simulink model "output_buffer"  (R2016b)
settings: Solver=VariableStepAuto  StartTime=0.0  StopTime=5000  RelTol=1e-3
undefined symbols (not defined in the file or in its folder): fft_stages, output_len_bits
libraries: xbsIndex_r4 x750, casper_library_misc x6, simulink x2
(part 3 of 3)

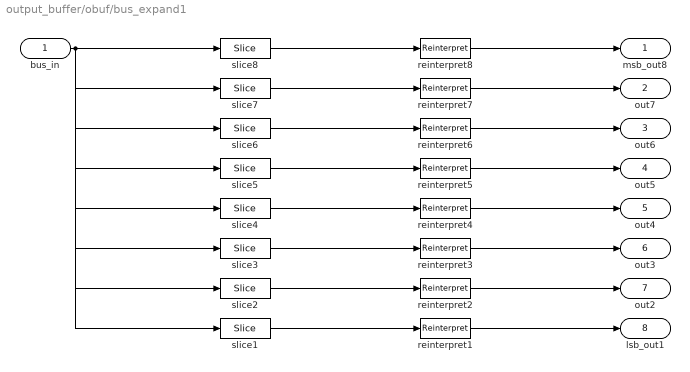
== system output_buffer/obuf/bus_expand1 ==
  bus_in : Inport
  reinterpret{1..8} (8 alike) : xbsIndex_r4/Reinterpret  force_arith_type=on  arith_type=Unsigned  force_bin_pt=on  bin_pt=0  block_type=reinterpret
  slice1 : xbsIndex_r4/Slice  nbits=32  boolean_output=off  mode=Upper Bit Location + Width  bit1=-224  base1=MSB of Input  bit0=0  base0=LSB of Input  dbl_ovrd=off  block_type=slice
  slice2 : xbsIndex_r4/Slice  nbits=32  boolean_output=off  mode=Upper Bit Location + Width  bit1=-192  base1=MSB of Input  bit0=0  base0=LSB of Input  dbl_ovrd=off  block_type=slice
  slice3 : xbsIndex_r4/Slice  nbits=32  boolean_output=off  mode=Upper Bit Location + Width  bit1=-160  base1=MSB of Input  bit0=0  base0=LSB of Input  dbl_ovrd=off  block_type=slice
  slice4 : xbsIndex_r4/Slice  nbits=32  boolean_output=off  mode=Upper Bit Location + Width  bit1=-128  base1=MSB of Input  bit0=0  base0=LSB of Input  dbl_ovrd=off  block_type=slice
  slice5 : xbsIndex_r4/Slice  nbits=32  boolean_output=off  mode=Upper Bit Location + Width  bit1=-96  base1=MSB of Input  bit0=0  base0=LSB of Input  dbl_ovrd=off  block_type=slice
  slice6 : xbsIndex_r4/Slice  nbits=32  boolean_output=off  mode=Upper Bit Location + Width  bit1=-64  base1=MSB of Input  bit0=0  base0=LSB of Input  dbl_ovrd=off  block_type=slice
  slice7 : xbsIndex_r4/Slice  nbits=32  boolean_output=off  mode=Upper Bit Location + Width  bit1=-32  base1=MSB of Input  bit0=0  base0=LSB of Input  dbl_ovrd=off  block_type=slice
  slice8 : xbsIndex_r4/Slice  nbits=32  boolean_output=off  mode=Upper Bit Location + Width  bit1=0  base1=MSB of Input  bit0=0  base0=LSB of Input  dbl_ovrd=off  block_type=slice
  msb_out8 : Outport
  out7 : Outport  Port=2
  out6 : Outport  Port=3
  out5 : Outport  Port=4
  out4 : Outport  Port=5
  out3 : Outport  Port=6
  out2 : Outport  Port=7
  lsb_out1 : Outport  Port=8
  wires:
  bus_in/1 -> slice8/1, slice7/1, slice6/1, slice5/1, slice4/1, slice3/1, slice2/1, slice1/1
  slice8/1 -> reinterpret8/1
  reinterpret8/1 -> msb_out8/1
  slice7/1 -> reinterpret7/1
  reinterpret7/1 -> out7/1
  slice6/1 -> reinterpret6/1
  reinterpret6/1 -> out6/1
  slice5/1 -> reinterpret5/1
  reinterpret5/1 -> out5/1
  slice4/1 -> reinterpret4/1
  reinterpret4/1 -> out4/1
  slice3/1 -> reinterpret3/1
  reinterpret3/1 -> out3/1
  slice2/1 -> reinterpret2/1
  reinterpret2/1 -> out2/1
  slice1/1 -> reinterpret1/1
  reinterpret1/1 -> lsb_out1/1

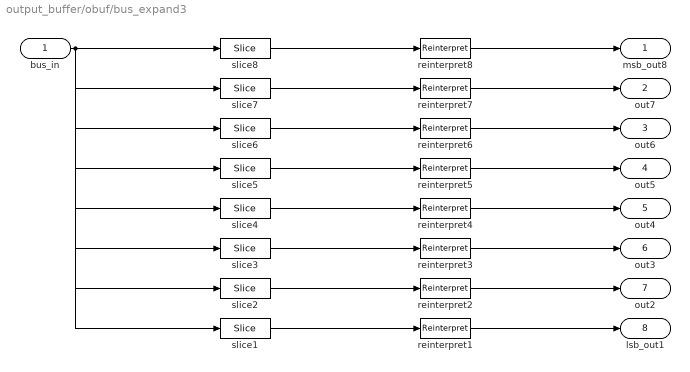
== system output_buffer/obuf/bus_expand3 ==
  bus_in : Inport
  reinterpret{1..8} (8 alike) : xbsIndex_r4/Reinterpret  force_arith_type=on  arith_type=Unsigned  force_bin_pt=on  bin_pt=0  block_type=reinterpret
  slice1 : xbsIndex_r4/Slice  nbits=32  boolean_output=off  mode=Upper Bit Location + Width  bit1=-224  base1=MSB of Input  bit0=0  base0=LSB of Input  dbl_ovrd=off  block_type=slice
  slice2 : xbsIndex_r4/Slice  nbits=32  boolean_output=off  mode=Upper Bit Location + Width  bit1=-192  base1=MSB of Input  bit0=0  base0=LSB of Input  dbl_ovrd=off  block_type=slice
  slice3 : xbsIndex_r4/Slice  nbits=32  boolean_output=off  mode=Upper Bit Location + Width  bit1=-160  base1=MSB of Input  bit0=0  base0=LSB of Input  dbl_ovrd=off  block_type=slice
  slice4 : xbsIndex_r4/Slice  nbits=32  boolean_output=off  mode=Upper Bit Location + Width  bit1=-128  base1=MSB of Input  bit0=0  base0=LSB of Input  dbl_ovrd=off  block_type=slice
  slice5 : xbsIndex_r4/Slice  nbits=32  boolean_output=off  mode=Upper Bit Location + Width  bit1=-96  base1=MSB of Input  bit0=0  base0=LSB of Input  dbl_ovrd=off  block_type=slice
  slice6 : xbsIndex_r4/Slice  nbits=32  boolean_output=off  mode=Upper Bit Location + Width  bit1=-64  base1=MSB of Input  bit0=0  base0=LSB of Input  dbl_ovrd=off  block_type=slice
  slice7 : xbsIndex_r4/Slice  nbits=32  boolean_output=off  mode=Upper Bit Location + Width  bit1=-32  base1=MSB of Input  bit0=0  base0=LSB of Input  dbl_ovrd=off  block_type=slice
  slice8 : xbsIndex_r4/Slice  nbits=32  boolean_output=off  mode=Upper Bit Location + Width  bit1=0  base1=MSB of Input  bit0=0  base0=LSB of Input  dbl_ovrd=off  block_type=slice
  msb_out8 : Outport
  out7 : Outport  Port=2
  out6 : Outport  Port=3
  out5 : Outport  Port=4
  out4 : Outport  Port=5
  out3 : Outport  Port=6
  out2 : Outport  Port=7
  lsb_out1 : Outport  Port=8
  wires:
  bus_in/1 -> slice8/1, slice7/1, slice6/1, slice5/1, slice4/1, slice3/1, slice2/1, slice1/1
  slice8/1 -> reinterpret8/1
  reinterpret8/1 -> msb_out8/1
  slice7/1 -> reinterpret7/1
  reinterpret7/1 -> out7/1
  slice6/1 -> reinterpret6/1
  reinterpret6/1 -> out6/1
  slice5/1 -> reinterpret5/1
  reinterpret5/1 -> out5/1
  slice4/1 -> reinterpret4/1
  reinterpret4/1 -> out4/1
  slice3/1 -> reinterpret3/1
  reinterpret3/1 -> out3/1
  slice2/1 -> reinterpret2/1
  reinterpret2/1 -> out2/1
  slice1/1 -> reinterpret1/1
  reinterpret1/1 -> lsb_out1/1

== system output_buffer/obuf/check_data_length ==
  dv : Inport
  data : Inport  Port=2
  Constant2 : xbsIndex_r4/Constant  const=255  gui_display_data_type=Fixed-point  arith_type=Unsigned  n_bits=9  bin_pt=0  preci_type=Single  exp_width=8  frac_width=24  explicit_period=on  period=1  equ=P=C  opselect=C  inp2=PCIN>>17  opr=+  inp1=P  carry=CIN  dbl_ovrd=off  block_type=constant
  Counter2 : xbsIndex_r4/Counter  cnt_type=Free Running  cnt_to=Inf  operation=Up  start_count=0  cnt_by_val=1  arith_type=Unsigned  n_bits=9  bin_pt=0  load_pin=off  rst=on  en=on  explicit_period=on  period=1  use_behavioral_HDL=off  implementation=Fabric  dbl_ovrd=off  block_type=counter
  Logical3 : xbsIndex_r4/Logical  logical_function=AND  inputs=2  en=off  latency=1  precision=Full  arith_type=Unsigned  n_bits=16  bin_pt=0  align_bp=on  dbl_ovrd=off  block_type=logical
  Logical4 : xbsIndex_r4/Logical  logical_function=AND  inputs=2  en=off  latency=1  precision=Full  arith_type=Unsigned  n_bits=16  bin_pt=0  align_bp=on  dbl_ovrd=off  block_type=logical
  Logical6 : xbsIndex_r4/Logical  logical_function=AND  inputs=2  en=off  latency=1  precision=Full  arith_type=Unsigned  n_bits=16  bin_pt=0  align_bp=on  dbl_ovrd=off  block_type=logical
  Register7 : xbsIndex_r4/Register  init=0  rst=off  en=on  dbl_ovrd=off  block_type=register
  Relational1 : xbsIndex_r4/Relational  mode=a=b  op_type=Bool  en=off  latency=0  dbl_ovrd=off  block_type=relational
  Relational2 : xbsIndex_r4/Relational  mode=a!=b  op_type=Bool  en=off  latency=0  dbl_ovrd=off  block_type=relational
  Relational3 : xbsIndex_r4/Relational  mode=a!=b  op_type=Bool  en=off  latency=0  dbl_ovrd=off  block_type=relational
  error : Outport
  wires:
  Constant2/1 -> Relational3/2
  data/1 -> Relational2/2, Relational1/2, Register7/1
  Logical6/1 -> error/1  "DLEN_ERROR"
  Relational2/1 -> Logical3/1
  Logical4/1 -> Counter2/2  "same"
  Logical3/1 -> Logical6/2, Counter2/1  "not_same"
  Relational3/1 -> Logical6/1
  dv/1 -> Logical3/2, Logical4/2, Register7/2
  Relational1/1 -> Logical4/1
  Counter2/1 -> Relational3/1  "data_len"
  Register7/1 -> Relational2/1, Relational1/1  "out_LASTdata"

== system output_buffer/obuf/edge_detect ==
  in : Inport
  Delay : xbsIndex_r4/Delay  rst=off  infoeditControl=Selection of Reset will increase slice count due to use of real FFs and instead of SRLs  en=off  latency=1  reg_retiming=off  dbl_ovrd=off  block_type=delay
      settings: xl_area=[0, 0, 0, 0, 0, 0, 0]
  Inverter : xbsIndex_r4/Inverter  en=off  latency=0  dbl_ovrd=off  block_type=inv
      settings: xl_area=[0, 0, 0, 0, 0, 0, 0]
  edge_op : xbsIndex_r4/Logical  logical_function=XNOR  inputs=2  en=off  latency=0  precision=Full  arith_type=Unsigned  n_bits=8  bin_pt=2  align_bp=on  dbl_ovrd=off  block_type=logical
      settings: xl_area=[0, 0, 0, 0, 0, 0, 0]
  out : Outport
  wires:
  Inverter/1 -> edge_op/1
  edge_op/1 -> out/1
  in/1 -> Inverter/1, Delay/1
  Delay/1 -> edge_op/2

== system output_buffer/obuf/error1 ==
  err : Inport
  armed : Inport  Port=2
  Gateway Out3 : xbsIndex_r4/Gateway Out  inherit_from_input=off  hdl_port=off  rows=1  columns=1  UseAsDAC=off  DACChannel='1'  interface=None  automatic_assignment=on  address_offset=hex2dec('00')  intf_name=''  intf_description=''  timing_constraint=None  locs_specified=off  LOCs={}  io_standard={}  block_type=gatewayout
  Logical : xbsIndex_r4/Logical  logical_function=OR  inputs=2  en=off  latency=1  precision=Full  arith_type=Unsigned  n_bits=16  bin_pt=0  align_bp=on  dbl_ovrd=off  block_type=logical
  Logical Operator2 : Logic  Operator=OR  AllPortsSameDT=off  OutDataTypeStr=boolean
  err_out : Outport
  wires:
  Logical/1 -> Gateway Out3/1
  armed/1 -> Logical/2
  err/1 -> Logical/1
  Logical Operator2/1 -> err_out/1
  [GLOBAL_ERR_WAIT] -> Logical Operator2/2
  Gateway Out3/1 -> Logical Operator2/1

== system output_buffer/obuf/error2 ==
  err : Inport
  armed : Inport  Port=2
  Gateway Out3 : xbsIndex_r4/Gateway Out  inherit_from_input=off  hdl_port=off  rows=1  columns=1  UseAsDAC=off  DACChannel='1'  interface=None  automatic_assignment=on  address_offset=hex2dec('00')  intf_name=''  intf_description=''  timing_constraint=None  locs_specified=off  LOCs={}  io_standard={}  block_type=gatewayout
  Logical : xbsIndex_r4/Logical  logical_function=OR  inputs=2  en=off  latency=1  precision=Full  arith_type=Unsigned  n_bits=16  bin_pt=0  align_bp=on  dbl_ovrd=off  block_type=logical
  Logical Operator2 : Logic  Operator=OR  AllPortsSameDT=off  OutDataTypeStr=boolean
  err_out : Outport
  wires:
  Gateway Out3/1 -> Logical Operator2/1
  [GLOBAL_ERR_WAIT] -> Logical Operator2/2
  Logical Operator2/1 -> err_out/1
  err/1 -> Logical/1
  armed/1 -> Logical/2
  Logical/1 -> Gateway Out3/1

== system output_buffer/obuf/error3 ==
  err : Inport
  armed : Inport  Port=2
  Gateway Out3 : xbsIndex_r4/Gateway Out  inherit_from_input=off  hdl_port=off  rows=1  columns=1  UseAsDAC=off  DACChannel='1'  interface=None  automatic_assignment=on  address_offset=hex2dec('00')  intf_name=''  intf_description=''  timing_constraint=None  locs_specified=off  LOCs={}  io_standard={}  block_type=gatewayout
  Logical : xbsIndex_r4/Logical  logical_function=OR  inputs=2  en=off  latency=1  precision=Full  arith_type=Unsigned  n_bits=16  bin_pt=0  align_bp=on  dbl_ovrd=off  block_type=logical
  Logical Operator2 : Logic  Operator=OR  AllPortsSameDT=off  OutDataTypeStr=boolean
  err_out : Outport
  wires:
  Gateway Out3/1 -> Logical Operator2/1
  [GLOBAL_ERR_WAIT] -> Logical Operator2/2
  Logical Operator2/1 -> err_out/1
  err/1 -> Logical/1
  armed/1 -> Logical/2
  Logical/1 -> Gateway Out3/1

== system output_buffer/obuf/error4 ==
  err : Inport
  armed : Inport  Port=2
  Gateway Out3 : xbsIndex_r4/Gateway Out  inherit_from_input=off  hdl_port=off  rows=1  columns=1  UseAsDAC=off  DACChannel='1'  interface=None  automatic_assignment=on  address_offset=hex2dec('00')  intf_name=''  intf_description=''  timing_constraint=None  locs_specified=off  LOCs={}  io_standard={}  block_type=gatewayout
  Logical : xbsIndex_r4/Logical  logical_function=OR  inputs=2  en=off  latency=1  precision=Full  arith_type=Unsigned  n_bits=16  bin_pt=0  align_bp=on  dbl_ovrd=off  block_type=logical
  Logical Operator2 : Logic  Operator=OR  AllPortsSameDT=off  OutDataTypeStr=boolean
  err_out : Outport
  wires:
  Logical/1 -> Gateway Out3/1
  armed/1 -> Logical/2
  err/1 -> Logical/1
  Logical Operator2/1 -> err_out/1
  [GLOBAL_ERR_WAIT] -> Logical Operator2/2
  Gateway Out3/1 -> Logical Operator2/1

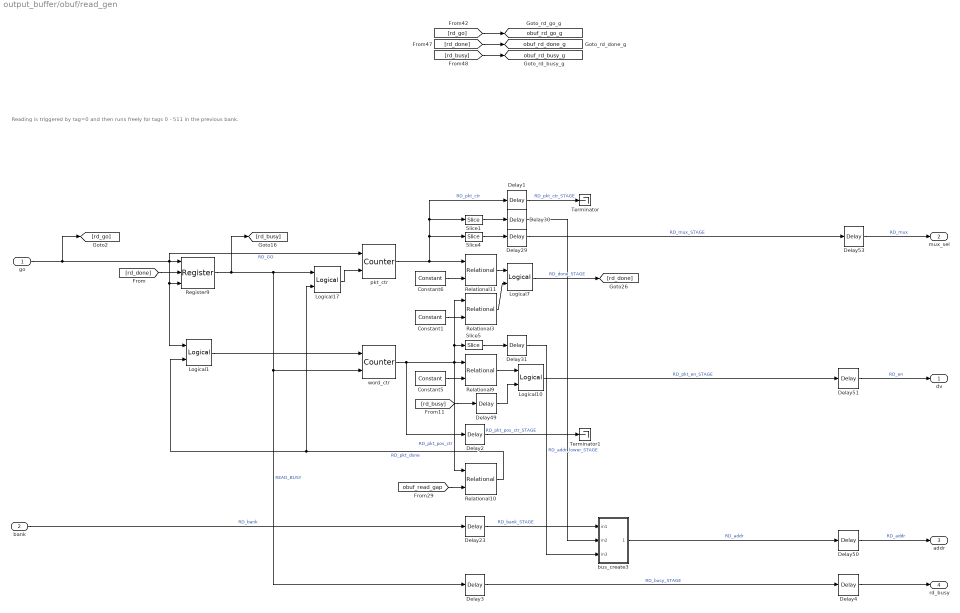
== system output_buffer/obuf/read_gen ==
  note: Reading is triggered by tag=0 and then runs freely for tags 0 - 511 in the previous bank.
  go : Inport
  bank : Inport  Port=2
  Constant1 : xbsIndex_r4/Constant  const=32  gui_display_data_type=Fixed-point  arith_type=Unsigned  n_bits=5  bin_pt=0  preci_type=Single  exp_width=8  frac_width=24  explicit_period=off  period=1  equ=P=C  opselect=C  inp2=PCIN>>17  opr=+  inp1=P  carry=CIN  dbl_ovrd=off  block_type=constant
  Constant5 : xbsIndex_r4/Constant  const=32  gui_display_data_type=Fixed-point  arith_type=Unsigned  n_bits=5  bin_pt=0  preci_type=Single  exp_width=8  frac_width=24  explicit_period=off  period=1  equ=P=C  opselect=C  inp2=PCIN>>17  opr=+  inp1=P  carry=CIN  dbl_ovrd=off  block_type=constant
  Constant6 : xbsIndex_r4/Constant  const=15  gui_display_data_type=Fixed-point  arith_type=Unsigned  n_bits=4  bin_pt=0  preci_type=Single  exp_width=8  frac_width=24  explicit_period=off  period=1  equ=P=C  opselect=C  inp2=PCIN>>17  opr=+  inp1=P  carry=CIN  dbl_ovrd=off  block_type=constant
  Delay{1..3,23,29..31,49} (8 alike) : xbsIndex_r4/Delay  rst=off  infoeditControl=Selection of Reset will increase slice count due to use of real FFs and instead of SRLs  en=off  latency=3  reg_retiming=off  dbl_ovrd=off  block_type=delay
      settings: infoedit=Hardware notes: A delay line is a chain, each link of which is an SRL16 or SRL32 followed by a flip-flop.
  Delay{4,50..51,53} (4 alike) : xbsIndex_r4/Delay  rst=off  infoeditControl=Selection of Reset will increase slice count due to use of real FFs and instead of SRLs  en=off  latency=1  reg_retiming=off  dbl_ovrd=off  block_type=delay
      settings: infoedit=Hardware notes: A delay line is a chain, each link of which is an SRL16 or SRL32 followed by a flip-flop.
  Logical1 : xbsIndex_r4/Logical  logical_function=OR  inputs=2  en=off  latency=0  precision=Full  arith_type=Unsigned  n_bits=16  bin_pt=0  align_bp=on  dbl_ovrd=off  block_type=logical
  Logical10 : xbsIndex_r4/Logical  logical_function=AND  inputs=2  en=off  latency=0  precision=Full  arith_type=Unsigned  n_bits=16  bin_pt=0  align_bp=on  dbl_ovrd=off  block_type=logical
  Logical17 : xbsIndex_r4/Logical  logical_function=AND  inputs=2  en=off  latency=0  precision=Full  arith_type=Unsigned  n_bits=16  bin_pt=0  align_bp=on  dbl_ovrd=off  block_type=logical
  Logical7 : xbsIndex_r4/Logical  logical_function=AND  inputs=2  en=off  latency=2  precision=Full  arith_type=Unsigned  n_bits=16  bin_pt=0  align_bp=on  dbl_ovrd=off  block_type=logical
  Register9 : xbsIndex_r4/Register  init=0  rst=on  en=on  dbl_ovrd=off  block_type=register
  Relational10 : xbsIndex_r4/Relational  mode=a=b  op_type=Bool  en=off  latency=3  dbl_ovrd=off  block_type=relational
  Relational11 : xbsIndex_r4/Relational  mode=a=b  op_type=Bool  en=off  latency=1  dbl_ovrd=off  block_type=relational
  Relational3 : xbsIndex_r4/Relational  mode=a=b  op_type=Bool  en=off  latency=1  dbl_ovrd=off  block_type=relational
  Relational9 : xbsIndex_r4/Relational  mode=a<=b  op_type=Bool  en=off  latency=3  dbl_ovrd=off  block_type=relational
  Slice1 : xbsIndex_r4/Slice  nbits=1  boolean_output=off  mode=Lower Bit Location + Width  bit1=0  base1=MSB of Input  bit0=3  base0=LSB of Input  dbl_ovrd=off  block_type=slice
  Slice4 : xbsIndex_r4/Slice  nbits=3  boolean_output=off  mode=Lower Bit Location + Width  bit1=0  base1=MSB of Input  bit0=0  base0=LSB of Input  dbl_ovrd=off  block_type=slice
  Slice5 : xbsIndex_r4/Slice  nbits=5  boolean_output=off  mode=Lower Bit Location + Width  bit1=0  base1=MSB of Input  bit0=0  base0=LSB of Input  dbl_ovrd=off  block_type=slice
  Terminator : Terminator
  Terminator1 : Terminator
  bus_create3 : Subsystem  AncestorBlock=casper_library_flow_control/bus_create  mask(bus_create){inputNum=3}
      mask prompts: inputNum "Number of inputs:"
      mask init:
      | bus_create_init(gcb,...
      |     'inputNum', inputNum);
  pkt_ctr : xbsIndex_r4/Counter  cnt_type=Free Running  cnt_to=Inf  operation=Up  start_count=0  cnt_by_val=1  arith_type=Unsigned  n_bits=4  bin_pt=0  load_pin=off  rst=on  en=on  explicit_period=on  period=1  use_behavioral_HDL=off  implementation=Fabric  dbl_ovrd=off  block_type=counter
  word_ctr : xbsIndex_r4/Counter  cnt_type=Free Running  cnt_to=Inf  operation=Up  start_count=0  cnt_by_val=1  arith_type=Unsigned  n_bits=6  bin_pt=0  load_pin=off  rst=on  en=on  explicit_period=on  period=1  use_behavioral_HDL=off  implementation=Fabric  dbl_ovrd=off  block_type=counter
  dv : Outport
  mux_sel : Outport  Port=2
  addr : Outport  Port=3
  rd_busy : Outport  Port=4
  tag scope: obuf_rd_busy_g=global, obuf_rd_done_g=global, obuf_rd_go_g=global
  wires:
  Delay50/1 -> addr/1  "RD_addr"
  Delay51/1 -> dv/1  "RD_en"
  go/1 -> pkt_ctr/1, Logical1/1, Register9/3, Register9/1, [rd_go]  "RD_GO"
  Delay23/1 -> bus_create3/1(in1)  "RD_bank_STAGE"
  bus_create3/1(bus_out) -> Delay50/1  "RD_addr"
  Constant1/1 -> Relational3/2
  Delay31/1 -> bus_create3/3(in3)  "RD_addr_lower_STAGE"
  Relational3/1 -> Logical7/2
  [rd_busy] -> Delay49/1
  Relational11/1 -> Logical7/1
  Slice5/1 -> Delay31/1
  Logical10/1 -> Delay51/1  "RD_pkt_en_STAGE"
  Delay53/1 -> mux_sel/1  "RD_mux"
  Slice1/1 -> Delay30/1
  Logical7/1 -> [rd_done]  "RD_done_STAGE"
  Relational9/1 -> Logical10/1
  Logical1/1 -> word_ctr/1
  Delay29/1 -> Delay53/1  "RD_mux_STAGE"
  Delay30/1 -> bus_create3/2(in2)
  Delay49/1 -> Logical10/2
  Register9/1 -> Logical17/1, Delay3/1, word_ctr/2, [rd_busy]  "READ_BUSY"
  pkt_ctr/1 -> Delay1/1, Slice1/1, Slice4/1, Relational11/1  "RD_pkt_ctr"
  Logical17/1 -> pkt_ctr/2
  Slice4/1 -> Delay29/1
  word_ctr/1 -> Delay2/1, Relational3/1, Slice5/1, Relational10/1, Relational9/1  "RD_pkt_pos_ctr"
  Constant5/1 -> Relational9/2
  [obuf_read_gap] -> Relational10/2
  Relational10/1 -> Logical17/2, Logical1/2  "RD_pkt_done"
  Constant6/1 -> Relational11/2
  bank/1 -> Delay23/1  "RD_bank"
  [rd_done] -> Register9/2
  [rd_go] -> [obuf_rd_go_g]
  [rd_done] -> [obuf_rd_done_g]
  [rd_busy] -> [obuf_rd_busy_g]
  Delay1/1 -> Terminator/1  "RD_pkt_ctr_STAGE"
  Delay2/1 -> Terminator1/1  "RD_pkt_pos_ctr_STAGE"
  Delay3/1 -> Delay4/1  "RD_busy_STAGE"
  Delay4/1 -> rd_busy/1

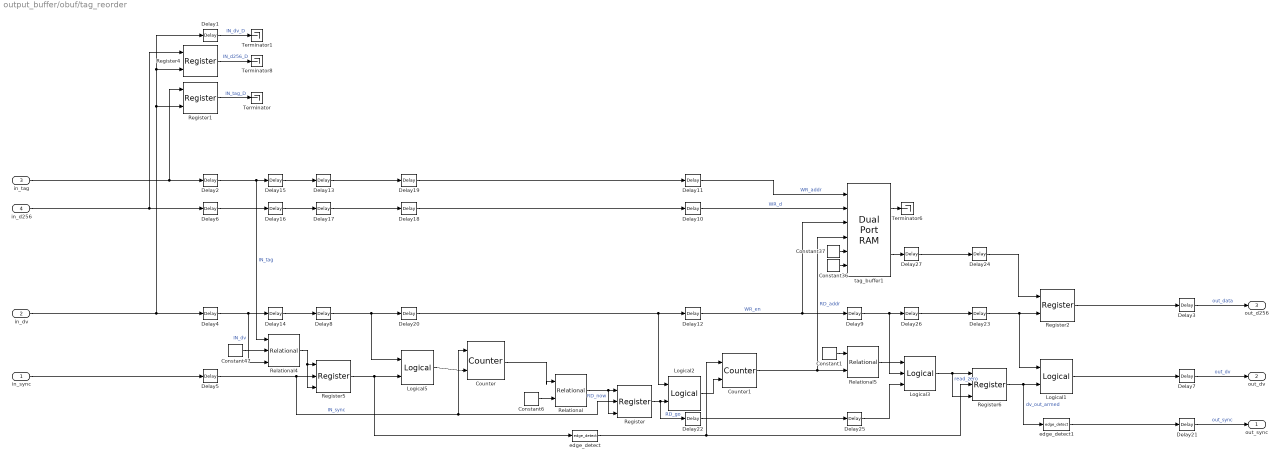
== system output_buffer/obuf/tag_reorder ==
  in_sync : Inport
  in_dv : Inport  Port=2
  in_tag : Inport  Port=3
  in_d256 : Inport  Port=4
  Constant1 : xbsIndex_r4/Constant  const=0  gui_display_data_type=Fixed-point  arith_type=Unsigned  n_bits=9  bin_pt=0  preci_type=Single  exp_width=8  frac_width=24  explicit_period=on  period=1  equ=P=C  opselect=C  inp2=PCIN>>17  opr=+  inp1=P  carry=CIN  dbl_ovrd=off  block_type=constant
  Constant36 : xbsIndex_r4/Constant  const=0  gui_display_data_type=Boolean  arith_type=Boolean  n_bits=16  bin_pt=14  preci_type=Single  exp_width=8  frac_width=24  explicit_period=on  period=1  equ=P=C  opselect=C  inp2=PCIN>>17  opr=+  inp1=P  carry=CIN  dbl_ovrd=off  block_type=constant
  Constant37 : xbsIndex_r4/Constant  const=0  gui_display_data_type=Fixed-point  arith_type=Unsigned  n_bits=256  bin_pt=0  preci_type=Single  exp_width=8  frac_width=24  explicit_period=on  period=1  equ=P=C  opselect=C  inp2=PCIN>>17  opr=+  inp1=P  carry=CIN  dbl_ovrd=off  block_type=constant
  Constant47 : xbsIndex_r4/Constant  const=0  gui_display_data_type=Fixed-point  arith_type=Unsigned  n_bits=9  bin_pt=0  preci_type=Single  exp_width=8  frac_width=24  explicit_period=on  period=1  equ=P=C  opselect=C  inp2=PCIN>>17  opr=+  inp1=P  carry=CIN  dbl_ovrd=off  block_type=constant
  Constant6 : xbsIndex_r4/Constant  const=250  gui_display_data_type=Fixed-point  arith_type=Unsigned  n_bits=9  bin_pt=0  preci_type=Single  exp_width=8  frac_width=24  explicit_period=on  period=1  equ=P=C  opselect=C  inp2=PCIN>>17  opr=+  inp1=P  carry=CIN  dbl_ovrd=off  block_type=constant
  Counter : xbsIndex_r4/Counter  cnt_type=Free Running  cnt_to=Inf  operation=Up  start_count=0  cnt_by_val=1  arith_type=Unsigned  n_bits=9  bin_pt=0  load_pin=off  rst=on  en=on  explicit_period=on  period=1  use_behavioral_HDL=off  implementation=Fabric  dbl_ovrd=off  block_type=counter
  Counter1 : xbsIndex_r4/Counter  cnt_type=Free Running  cnt_to=511  operation=Up  start_count=0  cnt_by_val=1  arith_type=Unsigned  n_bits=9  bin_pt=0  load_pin=off  rst=on  en=on  explicit_period=on  period=1  use_behavioral_HDL=off  implementation=Fabric  dbl_ovrd=off  block_type=counter
  Delay{1..2,4..6,8..20,22..27} (24 alike) : xbsIndex_r4/Delay  rst=off  infoeditControl=Selection of Reset will increase slice count due to use of real FFs and instead of SRLs  en=off  latency=1  reg_retiming=off  dbl_ovrd=off  block_type=delay
      settings: infoedit=Hardware notes: A delay line is a chain, each link of which is an SRL16 or SRL32 followed by a flip-flop.
  Delay21 : xbsIndex_r4/Delay  rst=off  infoeditControl=Selection of Reset will increase slice count due to use of real FFs and instead of SRLs  en=off  latency=0  reg_retiming=off  dbl_ovrd=off  block_type=delay
      settings: infoedit=Hardware notes: A delay line is a chain, each link of which is an SRL16 or SRL32 followed by a flip-flop.
  Delay3 : xbsIndex_r4/Delay  rst=off  infoeditControl=Selection of Reset will increase slice count due to use of real FFs and instead of SRLs  en=off  latency=0  reg_retiming=off  dbl_ovrd=off  block_type=delay
      settings: infoedit=Hardware notes: A delay line is a chain, each link of which is an SRL16 or SRL32 followed by a flip-flop.
  Delay7 : xbsIndex_r4/Delay  rst=off  infoeditControl=Selection of Reset will increase slice count due to use of real FFs and instead of SRLs  en=off  latency=0  reg_retiming=off  dbl_ovrd=off  block_type=delay
      settings: infoedit=Hardware notes: A delay line is a chain, each link of which is an SRL16 or SRL32 followed by a flip-flop.
  Logical1 : xbsIndex_r4/Logical  logical_function=AND  inputs=2  en=off  latency=1  precision=Full  arith_type=Unsigned  n_bits=16  bin_pt=0  align_bp=on  dbl_ovrd=off  block_type=logical
  Logical2 : xbsIndex_r4/Logical  logical_function=AND  inputs=2  en=off  latency=1  precision=Full  arith_type=Unsigned  n_bits=16  bin_pt=0  align_bp=on  dbl_ovrd=off  block_type=logical
  Logical3 : xbsIndex_r4/Logical  logical_function=AND  inputs=3  en=off  latency=1  precision=Full  arith_type=Unsigned  n_bits=16  bin_pt=0  align_bp=on  dbl_ovrd=off  block_type=logical
  Logical5 : xbsIndex_r4/Logical  logical_function=AND  inputs=2  en=off  latency=1  precision=Full  arith_type=Unsigned  n_bits=16  bin_pt=0  align_bp=on  dbl_ovrd=off  block_type=logical
  Register : xbsIndex_r4/Register  init=0  rst=on  en=on  dbl_ovrd=off  block_type=register
  Register1 : xbsIndex_r4/Register  init=0  rst=off  en=on  dbl_ovrd=off  block_type=register
  Register2 : xbsIndex_r4/Register  init=0  rst=off  en=on  dbl_ovrd=off  block_type=register
  Register4 : xbsIndex_r4/Register  init=0  rst=off  en=on  dbl_ovrd=off  block_type=register
  Register5 : xbsIndex_r4/Register  init=0  rst=on  en=on  dbl_ovrd=off  block_type=register
  Register6 : xbsIndex_r4/Register  init=0  rst=on  en=on  dbl_ovrd=off  block_type=register
  Relational : xbsIndex_r4/Relational  mode=a=b  op_type=Bool  en=off  latency=0  dbl_ovrd=off  block_type=relational
  Relational4 : xbsIndex_r4/Relational  mode=a=b  op_type=Bool  en=on  latency=1  dbl_ovrd=off  block_type=relational
  Relational5 : xbsIndex_r4/Relational  mode=a=b  op_type=Bool  en=off  latency=1  dbl_ovrd=off  block_type=relational
  Terminator{,1,6,8} (4 alike) : Terminator
  edge_detect : casper_library_misc/edge_detect  edge=Rising  polarity=Active High  x_in=[0 0.08 0.08 0.16 0.16 0.24 0.24 0.32 0.32 0.4]  y_in="[-1 -1  1  1  1  1  1  1  1  1]"  x_out=[0.6 0.68 0.68 0.76 0.76 0.84 0.84 0.92 0.92 1]  y_out="[-1 -1  1  1 -1 -1 -1 -1 -1 -1]"
  edge_detect1 : casper_library_misc/edge_detect  edge=Rising  polarity=Active High  x_in=[0 0.08 0.08 0.16 0.16 0.24 0.24 0.32 0.32 0.4]  y_in="[-1 -1  1  1  1  1  1  1  1  1]"  x_out=[0.6 0.68 0.68 0.76 0.76 0.84 0.84 0.92 0.92 1]  y_out="[-1 -1  1  1 -1 -1 -1 -1 -1 -1]"
  tag_buffer1 : xbsIndex_r4/Dual Port RAM  depth=512  initVector=zeros(1, 512)  distributed_mem=Block RAM  init_a=0  init_b=0  rst_a=off  rst_b=off  en_a=off  en_b=off  latency=1  write_mode_A=Read Before Write  write_mode_B=Read Before Write  optimize=Area  dbl_ovrd=off  block_type=dpram
  out_sync : Outport
  out_dv : Outport  Port=2
  out_d256 : Outport  Port=3
  wires:
  Delay14/1 -> Delay8/1
  Delay8/1 -> Delay20/1, Logical5/1
  Delay18/1 -> Delay10/1
  edge_detect/1 -> Counter1/1, Register6/2
  Register5/1 -> edge_detect/1, Logical5/2
  Delay17/1 -> Delay18/1
  Delay15/1 -> Delay13/1
  Delay19/1 -> Delay11/1
  Delay20/1 -> Logical2/1, Delay12/1
  Delay9/1 -> Logical3/2, Delay26/1
  Constant36/1 -> tag_buffer1/6
  Relational4/1 -> Register5/3, Register5/1
  in_d256/1 -> Delay6/1, Register4/1
  Constant47/1 -> Relational4/2
  Delay16/1 -> Delay17/1
  Delay12/1 -> tag_buffer1/3, Delay9/1  "WR_en"
  Delay13/1 -> Delay19/1
  Delay5/1 -> Counter/1, Register/2, Register5/2  "IN_sync"
  Register/1 -> Delay22/1, Logical2/2  "RD_go"
  Logical2/1 -> Counter1/2
  Register4/1 -> Terminator8/1  "IN_d256_D"
  Delay10/1 -> tag_buffer1/2  "WR_d"
  Logical5/1 -> Counter/2
  Delay6/1 -> Delay16/1
  Delay11/1 -> tag_buffer1/1  "WR_addr"
  tag_buffer1/1 -> Terminator6/1
  tag_buffer1/2 -> Delay27/1
  Constant37/1 -> tag_buffer1/5
  in_tag/1 -> Delay2/1, Register1/1
  in_dv/1 -> Delay4/1, Delay1/1, Register4/2, Register1/2
  Register1/1 -> Terminator/1  "IN_tag_D"
  Delay1/1 -> Terminator1/1  "IN_dv_D"
  Delay2/1 -> Relational4/1, Delay15/1  "IN_tag"
  in_sync/1 -> Delay5/1
  Delay4/1 -> Relational4/3, Delay14/1  "IN_dv"
  Counter/1 -> Relational/1
  Constant6/1 -> Relational/2
  Counter1/1 -> tag_buffer1/4, Relational5/2  "RD_addr"
  Relational/1 -> Register/3, Register/1  "RD_now"
  Constant1/1 -> Relational5/1
  Register6/1 -> edge_detect1/1, Logical1/2  "dv_out_armed"
  Delay3/1 -> out_d256/1  "out_data"
  Delay7/1 -> out_dv/1  "out_dv"
  Logical1/1 -> Delay7/1
  Register2/1 -> Delay3/1
  Delay23/1 -> Register2/2, Logical1/1
  Delay24/1 -> Register2/1
  edge_detect1/1 -> Delay21/1
  Delay21/1 -> out_sync/1  "out_sync"
  Relational5/1 -> Logical3/1
  Delay22/1 -> Delay25/1
  Delay26/1 -> Delay23/1
  Delay27/1 -> Delay24/1
  Logical3/1 -> Register6/3, Register6/1  "read_zero"
  Delay25/1 -> Logical3/3

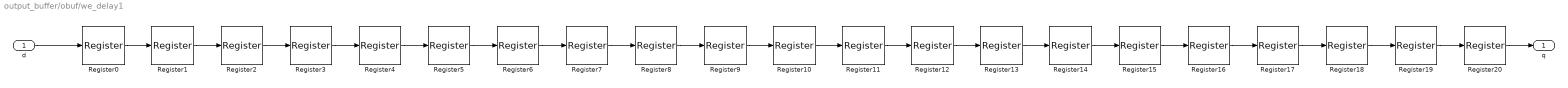
== system output_buffer/obuf/we_delay1 ==
  d : Inport
  Register{0..20} (21 alike) : xbsIndex_r4/Register  init=0  rst=off  en=off  dbl_ovrd=off  block_type=register
  q : Outport
  wires:
  Register20/1 -> q/1
  d/1 -> Register0/1
  Register19/1 -> Register20/1
  Register18/1 -> Register19/1
  Register17/1 -> Register18/1
  Register16/1 -> Register17/1
  Register15/1 -> Register16/1
  Register14/1 -> Register15/1
  Register13/1 -> Register14/1
  Register12/1 -> Register13/1
  Register11/1 -> Register12/1
  Register10/1 -> Register11/1
  Register9/1 -> Register10/1
  Register8/1 -> Register9/1
  Register7/1 -> Register8/1
  Register6/1 -> Register7/1
  Register5/1 -> Register6/1
  Register4/1 -> Register5/1
  Register3/1 -> Register4/1
  Register2/1 -> Register3/1
  Register1/1 -> Register2/1
  Register0/1 -> Register1/1

== system output_buffer/obuf/we_delay10 ==
  d : Inport
  Register{0..20} (21 alike) : xbsIndex_r4/Register  init=0  rst=off  en=off  dbl_ovrd=off  block_type=register
  q : Outport
  wires:
  Register0/1 -> Register1/1
  Register1/1 -> Register2/1
  Register2/1 -> Register3/1
  Register3/1 -> Register4/1
  Register4/1 -> Register5/1
  Register5/1 -> Register6/1
  Register6/1 -> Register7/1
  Register7/1 -> Register8/1
  Register8/1 -> Register9/1
  Register9/1 -> Register10/1
  Register10/1 -> Register11/1
  Register11/1 -> Register12/1
  Register12/1 -> Register13/1
  Register13/1 -> Register14/1
  Register14/1 -> Register15/1
  Register15/1 -> Register16/1
  Register16/1 -> Register17/1
  Register17/1 -> Register18/1
  Register18/1 -> Register19/1
  Register19/1 -> Register20/1
  d/1 -> Register0/1
  Register20/1 -> q/1

== system output_buffer/obuf/we_delay11 ==
  d : Inport
  Register{0..20} (21 alike) : xbsIndex_r4/Register  init=0  rst=off  en=off  dbl_ovrd=off  block_type=register
  q : Outport
  wires:
  Register0/1 -> Register1/1
  Register1/1 -> Register2/1
  Register2/1 -> Register3/1
  Register3/1 -> Register4/1
  Register4/1 -> Register5/1
  Register5/1 -> Register6/1
  Register6/1 -> Register7/1
  Register7/1 -> Register8/1
  Register8/1 -> Register9/1
  Register9/1 -> Register10/1
  Register10/1 -> Register11/1
  Register11/1 -> Register12/1
  Register12/1 -> Register13/1
  Register13/1 -> Register14/1
  Register14/1 -> Register15/1
  Register15/1 -> Register16/1
  Register16/1 -> Register17/1
  Register17/1 -> Register18/1
  Register18/1 -> Register19/1
  Register19/1 -> Register20/1
  d/1 -> Register0/1
  Register20/1 -> q/1

== system output_buffer/obuf/we_delay12 ==
  d : Inport
  Register{0..20} (21 alike) : xbsIndex_r4/Register  init=0  rst=off  en=off  dbl_ovrd=off  block_type=register
  q : Outport
  wires:
  Register20/1 -> q/1
  d/1 -> Register0/1
  Register19/1 -> Register20/1
  Register18/1 -> Register19/1
  Register17/1 -> Register18/1
  Register16/1 -> Register17/1
  Register15/1 -> Register16/1
  Register14/1 -> Register15/1
  Register13/1 -> Register14/1
  Register12/1 -> Register13/1
  Register11/1 -> Register12/1
  Register10/1 -> Register11/1
  Register9/1 -> Register10/1
  Register8/1 -> Register9/1
  Register7/1 -> Register8/1
  Register6/1 -> Register7/1
  Register5/1 -> Register6/1
  Register4/1 -> Register5/1
  Register3/1 -> Register4/1
  Register2/1 -> Register3/1
  Register1/1 -> Register2/1
  Register0/1 -> Register1/1

== system output_buffer/obuf/we_delay13 ==
  d : Inport
  Register{0..20} (21 alike) : xbsIndex_r4/Register  init=0  rst=off  en=off  dbl_ovrd=off  block_type=register
  q : Outport
  wires:
  Register0/1 -> Register1/1
  Register1/1 -> Register2/1
  Register2/1 -> Register3/1
  Register3/1 -> Register4/1
  Register4/1 -> Register5/1
  Register5/1 -> Register6/1
  Register6/1 -> Register7/1
  Register7/1 -> Register8/1
  Register8/1 -> Register9/1
  Register9/1 -> Register10/1
  Register10/1 -> Register11/1
  Register11/1 -> Register12/1
  Register12/1 -> Register13/1
  Register13/1 -> Register14/1
  Register14/1 -> Register15/1
  Register15/1 -> Register16/1
  Register16/1 -> Register17/1
  Register17/1 -> Register18/1
  Register18/1 -> Register19/1
  Register19/1 -> Register20/1
  d/1 -> Register0/1
  Register20/1 -> q/1

== system output_buffer/obuf/we_delay2 ==
  d : Inport
  Register{0..20} (21 alike) : xbsIndex_r4/Register  init=0  rst=off  en=off  dbl_ovrd=off  block_type=register
  q : Outport
  wires:
  Register0/1 -> Register1/1
  Register1/1 -> Register2/1
  Register2/1 -> Register3/1
  Register3/1 -> Register4/1
  Register4/1 -> Register5/1
  Register5/1 -> Register6/1
  Register6/1 -> Register7/1
  Register7/1 -> Register8/1
  Register8/1 -> Register9/1
  Register9/1 -> Register10/1
  Register10/1 -> Register11/1
  Register11/1 -> Register12/1
  Register12/1 -> Register13/1
  Register13/1 -> Register14/1
  Register14/1 -> Register15/1
  Register15/1 -> Register16/1
  Register16/1 -> Register17/1
  Register17/1 -> Register18/1
  Register18/1 -> Register19/1
  Register19/1 -> Register20/1
  d/1 -> Register0/1
  Register20/1 -> q/1

== system output_buffer/obuf/we_delay3 ==
  d : Inport
  Register{0..20} (21 alike) : xbsIndex_r4/Register  init=0  rst=off  en=off  dbl_ovrd=off  block_type=register
  q : Outport
  wires:
  Register20/1 -> q/1
  d/1 -> Register0/1
  Register19/1 -> Register20/1
  Register18/1 -> Register19/1
  Register17/1 -> Register18/1
  Register16/1 -> Register17/1
  Register15/1 -> Register16/1
  Register14/1 -> Register15/1
  Register13/1 -> Register14/1
  Register12/1 -> Register13/1
  Register11/1 -> Register12/1
  Register10/1 -> Register11/1
  Register9/1 -> Register10/1
  Register8/1 -> Register9/1
  Register7/1 -> Register8/1
  Register6/1 -> Register7/1
  Register5/1 -> Register6/1
  Register4/1 -> Register5/1
  Register3/1 -> Register4/1
  Register2/1 -> Register3/1
  Register1/1 -> Register2/1
  Register0/1 -> Register1/1

== system output_buffer/obuf/we_delay5 ==
  d : Inport
  Register{0..20} (21 alike) : xbsIndex_r4/Register  init=0  rst=off  en=off  dbl_ovrd=off  block_type=register
  q : Outport
  wires:
  Register0/1 -> Register1/1
  Register1/1 -> Register2/1
  Register2/1 -> Register3/1
  Register3/1 -> Register4/1
  Register4/1 -> Register5/1
  Register5/1 -> Register6/1
  Register6/1 -> Register7/1
  Register7/1 -> Register8/1
  Register8/1 -> Register9/1
  Register9/1 -> Register10/1
  Register10/1 -> Register11/1
  Register11/1 -> Register12/1
  Register12/1 -> Register13/1
  Register13/1 -> Register14/1
  Register14/1 -> Register15/1
  Register15/1 -> Register16/1
  Register16/1 -> Register17/1
  Register17/1 -> Register18/1
  Register18/1 -> Register19/1
  Register19/1 -> Register20/1
  d/1 -> Register0/1
  Register20/1 -> q/1

== system output_buffer/obuf/we_delay6 ==
  d : Inport
  Register{0..20} (21 alike) : xbsIndex_r4/Register  init=0  rst=off  en=off  dbl_ovrd=off  block_type=register
  q : Outport
  wires:
  Register20/1 -> q/1
  d/1 -> Register0/1
  Register19/1 -> Register20/1
  Register18/1 -> Register19/1
  Register17/1 -> Register18/1
  Register16/1 -> Register17/1
  Register15/1 -> Register16/1
  Register14/1 -> Register15/1
  Register13/1 -> Register14/1
  Register12/1 -> Register13/1
  Register11/1 -> Register12/1
  Register10/1 -> Register11/1
  Register9/1 -> Register10/1
  Register8/1 -> Register9/1
  Register7/1 -> Register8/1
  Register6/1 -> Register7/1
  Register5/1 -> Register6/1
  Register4/1 -> Register5/1
  Register3/1 -> Register4/1
  Register2/1 -> Register3/1
  Register1/1 -> Register2/1
  Register0/1 -> Register1/1

== system output_buffer/obuf/we_delay7 ==
  d : Inport
  Register{0..20} (21 alike) : xbsIndex_r4/Register  init=0  rst=off  en=off  dbl_ovrd=off  block_type=register
  q : Outport
  wires:
  Register20/1 -> q/1
  d/1 -> Register0/1
  Register19/1 -> Register20/1
  Register18/1 -> Register19/1
  Register17/1 -> Register18/1
  Register16/1 -> Register17/1
  Register15/1 -> Register16/1
  Register14/1 -> Register15/1
  Register13/1 -> Register14/1
  Register12/1 -> Register13/1
  Register11/1 -> Register12/1
  Register10/1 -> Register11/1
  Register9/1 -> Register10/1
  Register8/1 -> Register9/1
  Register7/1 -> Register8/1
  Register6/1 -> Register7/1
  Register5/1 -> Register6/1
  Register4/1 -> Register5/1
  Register3/1 -> Register4/1
  Register2/1 -> Register3/1
  Register1/1 -> Register2/1
  Register0/1 -> Register1/1

== system output_buffer/obuf/we_delay8 ==
  d : Inport
  Register{0..20} (21 alike) : xbsIndex_r4/Register  init=0  rst=off  en=off  dbl_ovrd=off  block_type=register
  q : Outport
  wires:
  Register0/1 -> Register1/1
  Register1/1 -> Register2/1
  Register2/1 -> Register3/1
  Register3/1 -> Register4/1
  Register4/1 -> Register5/1
  Register5/1 -> Register6/1
  Register6/1 -> Register7/1
  Register7/1 -> Register8/1
  Register8/1 -> Register9/1
  Register9/1 -> Register10/1
  Register10/1 -> Register11/1
  Register11/1 -> Register12/1
  Register12/1 -> Register13/1
  Register13/1 -> Register14/1
  Register14/1 -> Register15/1
  Register15/1 -> Register16/1
  Register16/1 -> Register17/1
  Register17/1 -> Register18/1
  Register18/1 -> Register19/1
  Register19/1 -> Register20/1
  d/1 -> Register0/1
  Register20/1 -> q/1

== system output_buffer/obuf/we_delay9 ==
  d : Inport
  Register{0..20} (21 alike) : xbsIndex_r4/Register  init=0  rst=off  en=off  dbl_ovrd=off  block_type=register
  q : Outport
  wires:
  Register20/1 -> q/1
  d/1 -> Register0/1
  Register19/1 -> Register20/1
  Register18/1 -> Register19/1
  Register17/1 -> Register18/1
  Register16/1 -> Register17/1
  Register15/1 -> Register16/1
  Register14/1 -> Register15/1
  Register13/1 -> Register14/1
  Register12/1 -> Register13/1
  Register11/1 -> Register12/1
  Register10/1 -> Register11/1
  Register9/1 -> Register10/1
  Register8/1 -> Register9/1
  Register7/1 -> Register8/1
  Register6/1 -> Register7/1
  Register5/1 -> Register6/1
  Register4/1 -> Register5/1
  Register3/1 -> Register4/1
  Register2/1 -> Register3/1
  Register1/1 -> Register2/1
  Register0/1 -> Register1/1

== system output_buffer/pktlen_check/edge_detect1 ==
  in : Inport
  Delay : xbsIndex_r4/Delay  rst=off  infoeditControl=Selection of Reset will increase slice count due to use of real FFs and instead of SRLs  en=off  latency=1  reg_retiming=off  dbl_ovrd=off  block_type=delay
      settings: xl_area=[0, 0, 0, 0, 0, 0, 0]
  Inverter : xbsIndex_r4/Inverter  en=off  latency=0  dbl_ovrd=off  block_type=inv
      settings: xl_area=[0, 0, 0, 0, 0, 0, 0]
  edge_op : xbsIndex_r4/Logical  logical_function=AND  inputs=2  en=off  latency=0  precision=Full  arith_type=Unsigned  n_bits=8  bin_pt=2  align_bp=on  dbl_ovrd=off  block_type=logical
      settings: xl_area=[0, 0, 0, 0, 0, 0, 0]
  out : Outport
  wires:
  Inverter/1 -> edge_op/1
  edge_op/1 -> out/1
  in/1 -> Inverter/1, Delay/1
  Delay/1 -> edge_op/2

== system output_buffer/obuf/read_gen/bus_create3 ==
  in1 : Inport
  in2 : Inport  Port=2
  in3 : Inport  Port=3
  concatenate : xbsIndex_r4/Concat  num_inputs=3  dbl_ovrd=off  block_type=concat
  reinterpret1 : xbsIndex_r4/Reinterpret  force_arith_type=on  arith_type=Unsigned  force_bin_pt=on  bin_pt=0  block_type=reinterpret
      settings: infoedit="Changes signal type without altering the binary representation.   You can changed the signal between signed and unsigned, and relocate the binary point.<br><br>Hardware notes: In hardware this block costs nothing.<br><br>Example:  Suppose the input is 6 bits wide, signed, with 2 fractional bits, and the output is forced to unsigned with 0 fractional bits.  Then an input of -2.0 (1110.00 in binary 2's complement) becomes an output of 56 (111000 in binary)."
  reinterpret2 : xbsIndex_r4/Reinterpret  force_arith_type=on  arith_type=Unsigned  force_bin_pt=on  bin_pt=0  block_type=reinterpret
      settings: infoedit="Changes signal type without altering the binary representation.   You can changed the signal between signed and unsigned, and relocate the binary point.<br><br>Hardware notes: In hardware this block costs nothing.<br><br>Example:  Suppose the input is 6 bits wide, signed, with 2 fractional bits, and the output is forced to unsigned with 0 fractional bits.  Then an input of -2.0 (1110.00 in binary 2's complement) becomes an output of 56 (111000 in binary)."
  reinterpret3 : xbsIndex_r4/Reinterpret  force_arith_type=on  arith_type=Unsigned  force_bin_pt=on  bin_pt=0  block_type=reinterpret
  bus_out : Outport
  wires:
  concatenate/1 -> bus_out/1
  in1/1 -> reinterpret1/1
  reinterpret1/1 -> concatenate/1
  in2/1 -> reinterpret2/1
  reinterpret2/1 -> concatenate/2
  in3/1 -> reinterpret3/1
  reinterpret3/1 -> concatenate/3
